simulink model "Prp"  (R2018a)
settings: configuration reference "cs_ert" (kept outside this file)
settings Model: DataDictionary=Prp.sldd  Creator=zhoutinglin  LastModifiedBy=zhoutinglin

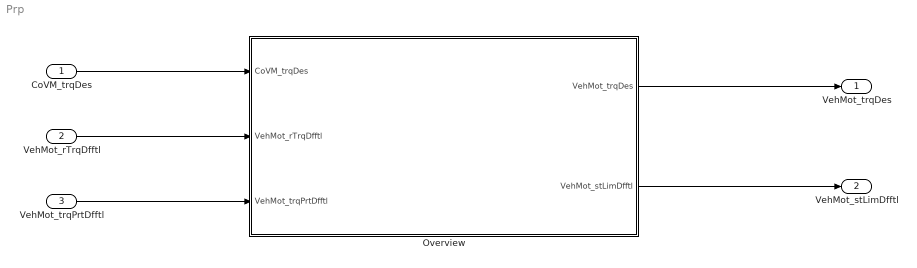
== system Prp ==
  CoVM_trqDes : Inport
  VehMot_rTrqDfftl : Inport  Port=2
  VehMot_trqPrtDfftl : Inport  Port=3
  Overview : Subsystem
  VehMot_trqDes : Outport
  VehMot_stLimDfftl : Outport  Port=2
  wires:
  CoVM_trqDes/1 -> Overview/1(CoVM_trqDes)
  VehMot_rTrqDfftl/1 -> Overview/2(VehMot_rTrqDfftl)
  VehMot_trqPrtDfftl/1 -> Overview/3(VehMot_trqPrtDfftl)
  Overview/1(VehMot_trqDes) -> VehMot_trqDes/1
  Overview/2(VehMot_stLimDfftl) -> VehMot_stLimDfftl/1

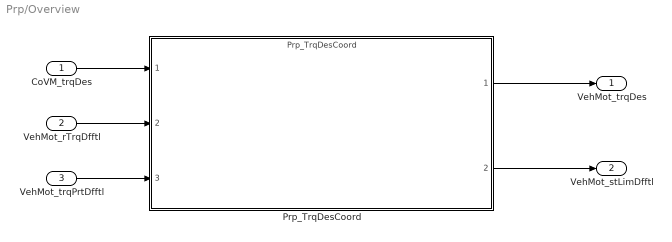
== system Prp/Overview ==
  CoVM_trqDes : Inport
  VehMot_rTrqDfftl : Inport  Port=2
  VehMot_trqPrtDfftl : Inport  Port=3
  Prp_TrqDesCoord : ModelReference  ModelNameDialog=Prp_TrqDesCoord  SimulationMode=Normal  ModelReferenceVersion=1.49
  VehMot_trqDes : Outport
  VehMot_stLimDfftl : Outport  Port=2
  wires:
  CoVM_trqDes/1 -> Prp_TrqDesCoord/1
  VehMot_rTrqDfftl/1 -> Prp_TrqDesCoord/2
  VehMot_trqPrtDfftl/1 -> Prp_TrqDesCoord/3
  Prp_TrqDesCoord/1 -> VehMot_trqDes/1
  Prp_TrqDesCoord/2 -> VehMot_stLimDfftl/1
